simulink library "takeoffToLanding_cl"  (R2018b)
settings: Solver=VariableStepAuto  StartTime=0.0  StopTime=10.0  RelTol=1e-3
undefined symbols (not defined in the file or in its folder): env, FLIGHTCONTROLLER, fltCtrl, initializeBussesFromBlock, maxDeflDns, maxDeflUps, TLSP, vhcl
libraries: filteredPIDController_ul x3, simulink x2, ctrlAllocMatrix_cl x2, dspsigops x1, eulAng2RotMat_ul x1, alphaBeta_ul x1, localApparentWind_ul x1, pathFollowingController_cl x1
settings Model: Creator=jldanie5  LastModifiedBy=jldanie5

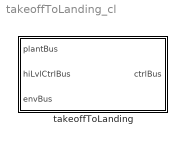
== system takeoffToLanding_cl ==
  takeoffToLanding : Subsystem  LoadFcn=initializeBussesFromBlock(gcb)  InitFcn=initializeBussesFromBlock(gcb)  StartFcn=initializeBussesFromBlock(gcb)  VariantControl=strcmpi(FLIGHTCONTROLLER,'takeoffToLanding')  mask{initPosForInitSStar=vhcl.initPosVecGnd.Value, fluidDensity=env.water.density.Value, pathCtrl=fltCtrl, aeroStruct=vhcl.struct('OCT.aeroSurf')}
      mask prompts: initPosForInitSStar "Initial Position"; fluidDensity "Fluid Density"; pathCtrl "Controller"; aeroStruct "Aerodynamic Structure"
      settings: MinAlgLoopOccurrences=on
      mask DialogControl Container3 Prompt: courseFollow Params
      mask DialogControl Container4 Prompt: setpointToOutput Params

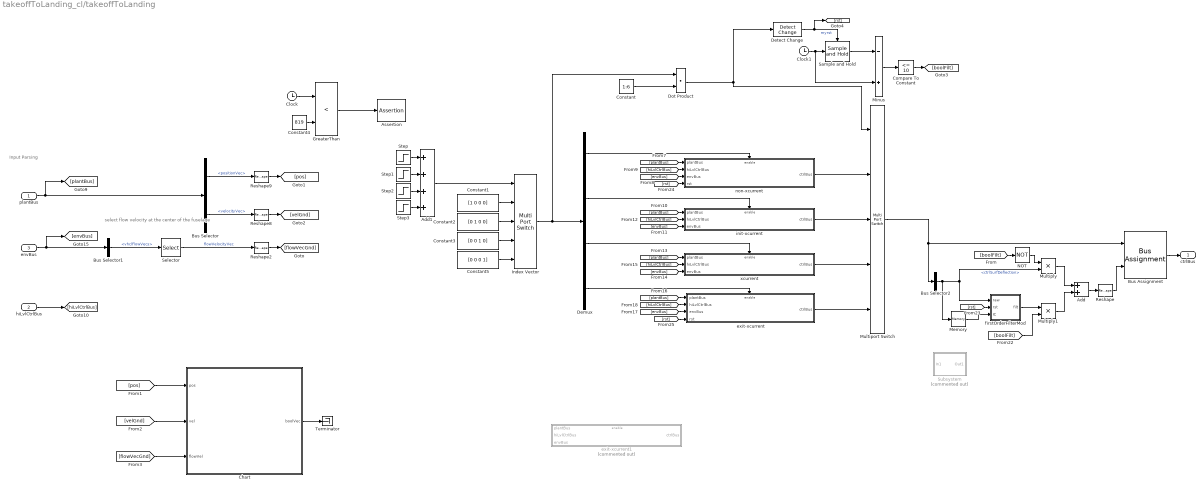
== system takeoffToLanding_cl/takeoffToLanding ==
  note: select flow velocity at the center of the fuselage
  note: Input Parsing
  plantBus : Inport  OutDataTypeStr=Bus: plantBus
  hiLvlCtrlBus : Inport  Port=2  OutDataTypeStr=Bus: hiLvlCtrlBus
  envBus : Inport  Port=3  OutDataTypeStr=Bus: envBus
  Add : Sum
  Add1 : Sum  Inputs=++++
  Assertion : Assertion  Enabled=off  AssertionFailFcn=set_param('OCTModel','SimulationCommand','pause')  StopWhenAssertionFail=off
  Bus Assignment : BusAssignment  AssignedSignals=ctrlSurfDeflection
  Bus Selector : BusSelector  OutputSignals=positionVec,velocityVec
  Bus Selector1 : BusSelector  OutputSignals=vhclFlowVecs
  Bus Selector2 : BusSelector  OutputSignals=ctrlSurfDeflection
  Chart : Stateflow chart  TreatAsAtomicUnit=on
  Clock : Clock
  Clock1 : Clock
  Compare To Constant : simulink/Logic and Bit Operations/Compare To Constant  relop=<=  const=10  OutDataTypeStr=boolean
  Constant : Constant  Value=1:6
  Constant1 : Constant  Value=[1 0 0 0]
  Constant2 : Constant  Value=[0 1 0 0]
  Constant3 : Constant  Value=[0 0 1 0]
  Constant4 : Constant  Value=819
  Constant5 : Constant  Value=[0 0 0 1]
  Demux : Demux
  Detect Change : simulink/Logic and Bit Operations/Detect Change  vinit=0  OutDataTypeStr=boolean
  Dot Product : DotProduct  InputSameDT=on  OutDataTypeStr=Inherit: Inherit via internal rule
  GreaterThan : RelationalOperator  Operator=<  OutDataTypeStr=boolean  RndMeth=Simplest
  Index Vector : MultiPortSwitch  DataPortOrder=Zero-based contiguous  Inputs=4  zeroidx=on
  Memory : Memory  InitialCondition=[0;0;0;0]
  Minus : Sum  Inputs=-+
  Multiply : Product
  Multiply1 : Product
  Multiport Switch : MultiPortSwitch  Inputs=4  DataPortIndices={1,2,3,4,5,6}  DiagnosticForDefault=Warning
  NOT : Logic  Operator=NOT  IconShape=distinctive  AllPortsSameDT=off  OutDataTypeStr=boolean
  Reshape : Reshape
  Reshape2 : Reshape  OutputDimensionality=Column vector (2-D)
  Reshape8 : Reshape  OutputDimensionality=Column vector (2-D)
  Reshape9 : Reshape  OutputDimensionality=Column vector (2-D)
  Sample and Hold : dspsigops/Sample and Hold  trig=Rising edge  initCond=0  latchinput=off
  Selector : Selector  NumberOfDimensions=2  InputPortWidth=3  IndexOptions=Select all,Index vector (dialog)  Indices=[1 3],5  OutputSizes=1,1
  Step : Step  Time=500  SampleTime=0
  Step1 : Step  Time=510  SampleTime=0
  Step2 : Step  Time=800  SampleTime=0
  Step3 : Step  Time=820  After=-3  SampleTime=0
  Subsystem : Subsystem  Commented=on
  Terminator : Terminator
  exit-xcurrent : Subsystem  TreatAsAtomicUnit=on
  exit-xcurrent1 : Subsystem  Commented=on  TreatAsAtomicUnit=on
  "firstOrderFilterMod " : Subsystem  TreatAsAtomicUnit=on  mask{tau=1, ic=0}
      mask prompts: tau "Time Const [s]"; ic "Initial Condition"
      settings: MinAlgLoopOccurrences=on
  init-xcurrent : Subsystem  TreatAsAtomicUnit=on
  non-xcurrent : Subsystem  TreatAsAtomicUnit=on
  xcurrent : Subsystem  TreatAsAtomicUnit=on
  ctrlBus : Outport  OutDataTypeStr=Bus: fltCtrlBus
  wires:
  Constant5/1 -> Index Vector/5
  plantBus/1 -> [plantBus], Bus Selector/1
  Bus Selector/2 -> Reshape8/1  "<velocityVec>"
  Bus Selector/1 -> Reshape9/1  "<positionVec>"
  Reshape2/1 -> [flowVecGnd]
  Reshape8/1 -> [velGnd]
  Reshape9/1 -> [pos]
  Selector/1 -> Reshape2/1  "flowVelocityVec"
  envBus/1 -> [envBus], Bus Selector1/1
  Bus Selector1/1 -> Selector/1  "<vhclFlowVecs>"
  [pos] -> Chart/1(pos)
  [velGnd] -> Chart/2(vel)
  [flowVecGnd] -> Chart/3(flowVel)
  [envBus] -> non-xcurrent/3(envBus)
  [plantBus] -> non-xcurrent/1(plantBus)
  [hiLvlCtrlBus] -> non-xcurrent/2(hiLvlCtrlBus)
  [hiLvlCtrlBus] -> xcurrent/2(hiLvlCtrlBus)
  [plantBus] -> xcurrent/1(plantBus)
  [envBus] -> xcurrent/3(envBus)
  [hiLvlCtrlBus] -> init-xcurrent/2(hiLvlCtrlBus)
  [envBus] -> init-xcurrent/3(envBus)
  [plantBus] -> init-xcurrent/1(plantBus)
  [plantBus] -> exit-xcurrent/1(plantBus)
  [envBus] -> exit-xcurrent/3(envBus)
  [hiLvlCtrlBus] -> exit-xcurrent/2(hiLvlCtrlBus)
  Constant/1 -> Dot Product/2
  Dot Product/1 -> Multiport Switch/1, Detect Change/1
  Chart/1(boolVec) -> Terminator/1
  hiLvlCtrlBus/1 -> [hiLvlCtrlBus]
  Constant1/1 -> Index Vector/2
  Constant2/1 -> Index Vector/3
  Constant3/1 -> Index Vector/4
  Clock/1 -> GreaterThan/1
  Constant4/1 -> GreaterThan/2
  GreaterThan/1 -> Assertion/1
  Add1/1 -> Index Vector/1
  Index Vector/1 -> Dot Product/1, Demux/1
  Clock1/1 -> Minus/2, Sample and Hold/1
  Detect Change/1 -> [rst], Sample and Hold/Trigger  "myrst"
  Sample and Hold/1 -> Minus/1
  Minus/1 -> Compare To Constant/1
  Compare To Constant/1 -> [boolFilt]
  Bus Assignment/1 -> ctrlBus/1
  Multiport Switch/1 -> Bus Selector2/1, Bus Assignment/1
  Bus Selector2/1 -> Multiply/2, "firstOrderFilterMod "/1(raw), Memory/1  "<ctrlSurfDeflection>"
  [boolFilt] -> NOT/1
  NOT/1 -> Multiply/1
  "firstOrderFilterMod "/1(filt) -> Multiply1/1
  [boolFilt] -> Multiply1/2
  [rst] -> "firstOrderFilterMod "/2(rst)
  Multiply/1 -> Add/1
  Multiply1/1 -> Add/2
  Add/1 -> Reshape/1
  Reshape/1 -> Bus Assignment/2
  Memory/1 -> "firstOrderFilterMod "/3(IC)
  Step/1 -> Add1/1
  Step1/1 -> Add1/2
  Step2/1 -> Add1/3
  Step3/1 -> Add1/4
  [rst] -> non-xcurrent/4("rst ")
  [rst] -> exit-xcurrent/4(rst)
  exit-xcurrent/1(ctrlBus) -> Multiport Switch/5
  xcurrent/1(ctrlBus) -> Multiport Switch/4
  init-xcurrent/1(ctrlBus) -> Multiport Switch/3
  non-xcurrent/1(ctrlBus) -> Multiport Switch/2
  Demux/1 -> non-xcurrent/Enable
  Demux/2 -> init-xcurrent/Enable
  Demux/3 -> xcurrent/Enable
  Demux/4 -> exit-xcurrent/Enable

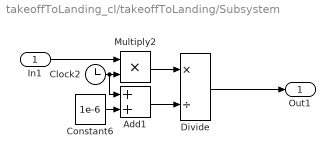
== system takeoffToLanding_cl/takeoffToLanding/Subsystem ==
  In1 : Inport
  Add1 : Sum
  Clock2 : Clock
  Constant6 : Constant  Value=1e-6
  Divide : Product  Inputs=*/
  Multiply2 : Product
  Out1 : Outport
  wires:
  In1/1 -> Multiply2/1
  Constant6/1 -> Add1/2
  Clock2/1 -> Add1/1, Multiply2/2
  Divide/1 -> Out1/1
  Multiply2/1 -> Divide/1
  Add1/1 -> Divide/2

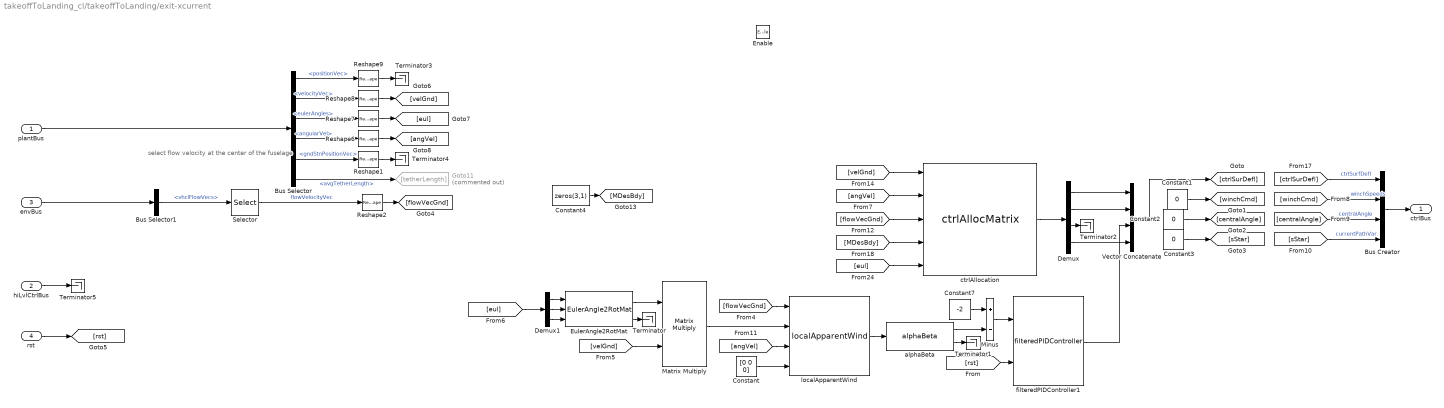
== system takeoffToLanding_cl/takeoffToLanding/exit-xcurrent ==
  note: select flow velocity at the center of the fuselage
  plantBus : Inport  OutDataTypeStr=Bus: plantBus
  hiLvlCtrlBus : Inport  Port=2  OutDataTypeStr=Bus: hiLvlCtrlBus
  envBus : Inport  Port=3  OutDataTypeStr=Bus: envBus
  rst : Inport  Port=4
  Enable : EnablePort
  Bus Creator : BusCreator  Inputs=4  OutDataTypeStr=Bus: fltCtrlBus
      settings: InheritFromInputs=off
  Bus Selector : BusSelector  OutputSignals=positionVec,velocityVec,eulerAngles,angularVel,gndStnPositionVec,avgTetherLength
  Bus Selector1 : BusSelector  OutputSignals=vhclFlowVecs
  Constant : Constant  Value=[0 0 0]
  Constant1 : Constant  Value=0
  Constant2 : Constant  Value=0
  Constant3 : Constant  Value=0
  Constant4 : Constant  Value=zeros(3,1)
  Constant7 : Constant  Value=-2
  Demux : Demux
  Demux1 : Demux  Outputs=3
  EulerAngle2RotMat : eulAng2RotMat_ul/EulerAngle2RotMat  SystemSampleTime=-1
  Goto11 : Goto  Commented=on  GotoTag=tetherLength
  Matrix Multiply : Product  Multiplication=Matrix(*)
  Minus : Sum  Inputs=+-
  Reshape{1..2,6..9} (6 alike) : Reshape  OutputDimensionality=Column vector (2-D)
  Selector : Selector  NumberOfDimensions=2  InputPortWidth=3  IndexOptions=Select all,Index vector (dialog)  Indices=[1 3],5  OutputSizes=1,1
  Terminator{,1..5} (6 alike) : Terminator
  Vector Concatenate : Concatenate  NumInputs=4
  alphaBeta : alphaBeta_ul/alphaBeta  SystemSampleTime=-1
  ctrlAllocation : ctrlAllocMatrix_cl/ctrlAllocMatrix  aeroStruct=aeroStruct  fluidDensity=fluidDensity  ctrlUpMax=pathCtrl.controlSigMax.upperLimit.Value  ctrlDnMax=pathCtrl.controlSigMax.lowerLimit.Value
  filteredPIDController1 : filteredPIDController_ul/filteredPIDController  kp=kpElev  ki=kiElev  kd=kdElev  Value=.01  externalReset=rising
  localApparentWind : localApparentWind_ul/localApparentWind  SystemSampleTime=-1
  ctrlBus : Outport  OutDataTypeStr=Bus: fltCtrlBus
  wires:
  [sStar] -> Bus Creator/4  "currentPathVar"
  [ctrlSurDefl] -> Bus Creator/1  "ctrlSurfDefl"
  [winchCmd] -> Bus Creator/2  "winchSpeeds"
  Bus Creator/1 -> ctrlBus/1
  [centralAngle] -> Bus Creator/3  "centralAngle"
  Constant1/1 -> [winchCmd]
  Constant2/1 -> [centralAngle]
  Constant3/1 -> [sStar]
  Bus Selector/1 -> Reshape9/1  "<positionVec>"
  Bus Selector/3 -> Reshape7/1  "<eulerAngles>"
  Bus Selector/2 -> Reshape8/1  "<velocityVec>"
  Reshape7/1 -> [eul]
  Bus Selector/4 -> Reshape6/1  "<angularVel>"
  Reshape8/1 -> [velGnd]
  Selector/1 -> Reshape2/1  "flowVelocityVec"
  Reshape9/1 -> Terminator3/1
  Bus Selector/5 -> Reshape1/1  "<gndStnPositionVec>"
  Reshape2/1 -> [flowVecGnd]
  Bus Selector1/1 -> Selector/1  "<vhclFlowVecs>"
  envBus/1 -> Bus Selector1/1
  Reshape1/1 -> Terminator4/1
  plantBus/1 -> Bus Selector/1
  Reshape6/1 -> [angVel]
  [flowVecGnd] -> ctrlAllocation/3
  [angVel] -> ctrlAllocation/2
  [eul] -> ctrlAllocation/5
  [MDesBdy] -> ctrlAllocation/4
  [velGnd] -> ctrlAllocation/1
  Bus Selector/6 -> Goto11/1  "<avgTetherLength>"
  ctrlAllocation/1 -> Demux/1
  Vector Concatenate/1 -> [ctrlSurDefl]
  Minus/1 -> filteredPIDController1/1
  Demux/1 -> Vector Concatenate/1
  Demux/2 -> Vector Concatenate/2
  Demux/4 -> Vector Concatenate/4
  localApparentWind/1 -> alphaBeta/1
  [flowVecGnd] -> localApparentWind/1
  Demux1/1 -> EulerAngle2RotMat/1
  Demux1/2 -> EulerAngle2RotMat/2
  Demux1/3 -> EulerAngle2RotMat/3
  [eul] -> Demux1/1
  EulerAngle2RotMat/1 -> Matrix Multiply/1
  [velGnd] -> Matrix Multiply/2
  EulerAngle2RotMat/2 -> Terminator/1
  Matrix Multiply/1 -> localApparentWind/2
  [angVel] -> localApparentWind/3
  Constant/1 -> localApparentWind/4
  Constant7/1 -> Minus/1
  alphaBeta/1 -> Minus/2
  filteredPIDController1/1 -> Vector Concatenate/3
  Demux/3 -> Terminator2/1
  alphaBeta/2 -> Terminator1/1
  Constant4/1 -> [MDesBdy]
  hiLvlCtrlBus/1 -> Terminator5/1
  rst/1 -> [rst]
  [rst] -> filteredPIDController1/2

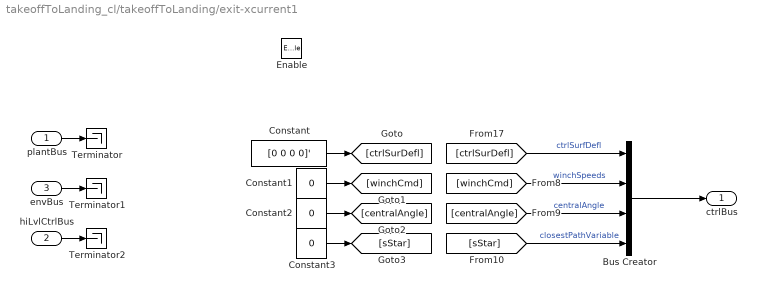
== system takeoffToLanding_cl/takeoffToLanding/exit-xcurrent1 ==
  plantBus : Inport  OutDataTypeStr=Bus: plantBus
  hiLvlCtrlBus : Inport  Port=2  OutDataTypeStr=Bus: hiLvlCtrlBus
  envBus : Inport  Port=3  OutDataTypeStr=Bus: envBus
  Enable : EnablePort
  Bus Creator : BusCreator  Inputs=4  OutDataTypeStr=Bus: fltCtrlBus
      settings: InheritFromInputs=off
  Constant : Constant  Value=[0 0 0 0]'
  Constant1 : Constant  Value=0
  Constant2 : Constant  Value=0
  Constant3 : Constant  Value=0
  Terminator : Terminator
  Terminator1 : Terminator
  Terminator2 : Terminator
  ctrlBus : Outport  OutDataTypeStr=Bus: fltCtrlBus
  wires:
  [ctrlSurDefl] -> Bus Creator/1  "ctrlSurfDefl"
  [centralAngle] -> Bus Creator/3  "centralAngle"
  [winchCmd] -> Bus Creator/2  "winchSpeeds"
  envBus/1 -> Terminator1/1
  hiLvlCtrlBus/1 -> Terminator2/1
  Constant2/1 -> [centralAngle]
  plantBus/1 -> Terminator/1
  [sStar] -> Bus Creator/4  "closestPathVariable"
  Constant1/1 -> [winchCmd]
  Bus Creator/1 -> ctrlBus/1
  Constant3/1 -> [sStar]
  Constant/1 -> [ctrlSurDefl]

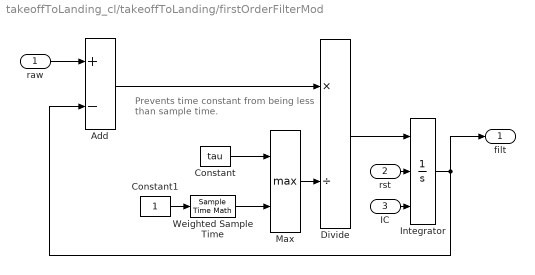
== system takeoffToLanding_cl/takeoffToLanding/firstOrderFilterMod  ==
  note: Prevents time constant from
      | being less than sample time.
  raw : Inport
  rst : Inport  Port=2
  IC : Inport  Port=3
  Add : Sum  Inputs=+-
  Constant : Constant  Value=tau
  Constant1 : Constant
  Divide : Product  Inputs=*/
  Integrator : Integrator  ExternalReset=rising  InitialConditionSource=external  InitialCondition=ic
  Max : MinMax  Function=max  Inputs=2
  Weighted Sample Time : SampleTimeMath  TsampMathOp=Ts Only
  filt : Outport
  wires:
  raw/1 -> Add/1
  Add/1 -> Divide/1
  Max/1 -> Divide/2
  Constant/1 -> Max/1
  Constant1/1 -> Weighted Sample Time/1
  Weighted Sample Time/1 -> Max/2
  Divide/1 -> Integrator/1
  Integrator/1 -> Add/2, filt/1
  IC/1 -> Integrator/3
  rst/1 -> Integrator/2

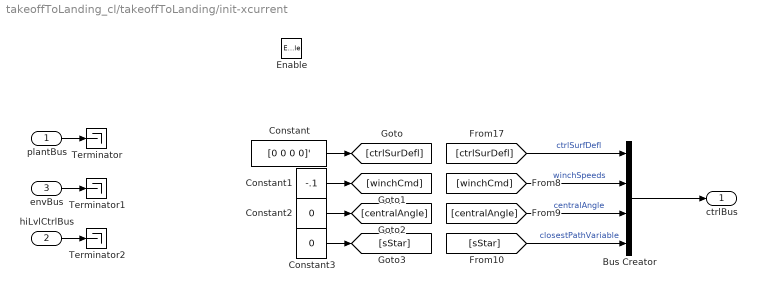
== system takeoffToLanding_cl/takeoffToLanding/init-xcurrent ==
  plantBus : Inport  OutDataTypeStr=Bus: plantBus
  hiLvlCtrlBus : Inport  Port=2  OutDataTypeStr=Bus: hiLvlCtrlBus
  envBus : Inport  Port=3  OutDataTypeStr=Bus: envBus
  Enable : EnablePort
  Bus Creator : BusCreator  Inputs=4  OutDataTypeStr=Bus: fltCtrlBus
      settings: InheritFromInputs=off
  Constant : Constant  Value=[0 0 0 0]'
  Constant1 : Constant  Value=-.1
  Constant2 : Constant  Value=0
  Constant3 : Constant  Value=0
  Terminator : Terminator
  Terminator1 : Terminator
  Terminator2 : Terminator
  ctrlBus : Outport  OutDataTypeStr=Bus: fltCtrlBus
  wires:
  [ctrlSurDefl] -> Bus Creator/1  "ctrlSurfDefl"
  [centralAngle] -> Bus Creator/3  "centralAngle"
  [winchCmd] -> Bus Creator/2  "winchSpeeds"
  envBus/1 -> Terminator1/1
  hiLvlCtrlBus/1 -> Terminator2/1
  Constant2/1 -> [centralAngle]
  plantBus/1 -> Terminator/1
  [sStar] -> Bus Creator/4  "closestPathVariable"
  Constant1/1 -> [winchCmd]
  Bus Creator/1 -> ctrlBus/1
  Constant3/1 -> [sStar]
  Constant/1 -> [ctrlSurDefl]

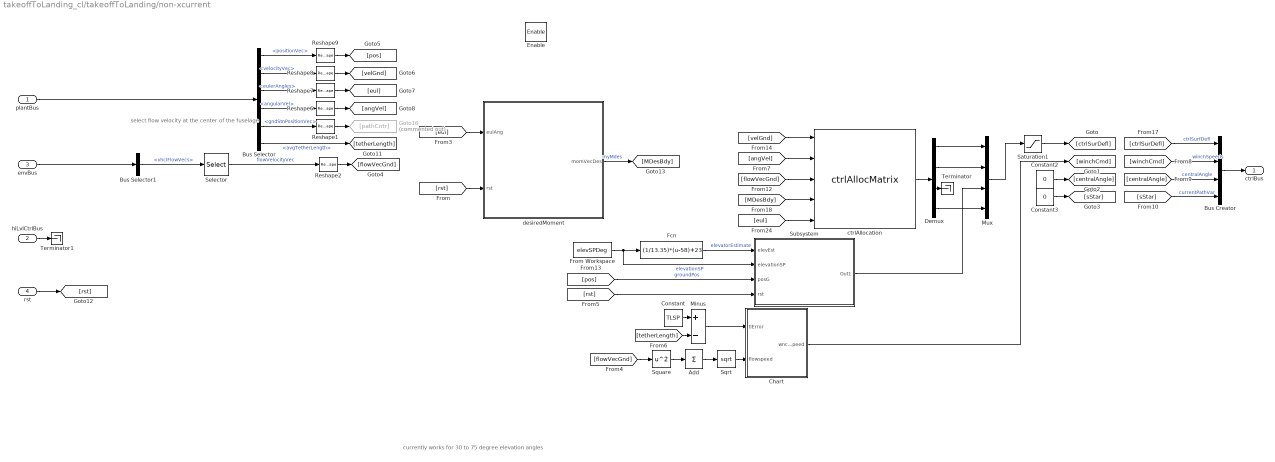
== system takeoffToLanding_cl/takeoffToLanding/non-xcurrent ==
  note: select flow velocity at the center of the fuselage
  note: currently works for 30 to 75 degree elevation angles
  plantBus : Inport  OutDataTypeStr=Bus: plantBus
  hiLvlCtrlBus : Inport  Port=2  OutDataTypeStr=Bus: hiLvlCtrlBus
  envBus : Inport  Port=3  OutDataTypeStr=Bus: envBus
  "rst " : Inport  Port=4
  Enable : EnablePort
  Add : Sum  Inputs=+
  Bus Creator : BusCreator  Inputs=4  OutDataTypeStr=Bus: fltCtrlBus
      settings: InheritFromInputs=off
  Bus Selector : BusSelector  OutputSignals=positionVec,velocityVec,eulerAngles,angularVel,gndStnPositionVec,avgTetherLength
  Bus Selector1 : BusSelector  OutputSignals=vhclFlowVecs
  Chart : Stateflow chart  TreatAsAtomicUnit=on
  Constant : Constant  Value=TLSP
  Constant2 : Constant  Value=0
  Constant3 : Constant  Value=0
  Demux : Demux
  Fcn : Fcn  Expr=(1/13.35)*(u-58)+23
  From Workspace : FromWorkspace  VariableName=elevSPDeg  SampleTime=0
  Goto16 : Goto  Commented=on  GotoTag=pathCntr
  Minus : Sum  Inputs=+-
  Mux : Mux
  Reshape{1..2,6..9} (6 alike) : Reshape  OutputDimensionality=Column vector (2-D)
  Saturation1 : Saturate  UpperLimit=maxDeflUps  LowerLimit=maxDeflDns
  Selector : Selector  NumberOfDimensions=2  InputPortWidth=3  IndexOptions=Select all,Index vector (dialog)  Indices=[1 3],5  OutputSizes=1,1
  Sqrt : Sqrt  SaturateOnIntegerOverflow=on
  Square : Math  Operator=square  SaturateOnIntegerOverflow=on
  Subsystem : Subsystem
  Terminator : Terminator
  Terminator1 : Terminator
  ctrlAllocation : ctrlAllocMatrix_cl/ctrlAllocMatrix  aeroStruct=aeroStruct  fluidDensity=fluidDensity  ctrlUpMax=pathCtrl.controlSigMax.upperLimit.Value  ctrlDnMax=pathCtrl.controlSigMax.lowerLimit.Value
  desiredMoment : Subsystem
  ctrlBus : Outport  OutDataTypeStr=Bus: fltCtrlBus
  wires:
  [sStar] -> Bus Creator/4  "currentPathVar"
  [ctrlSurDefl] -> Bus Creator/1  "ctrlSurfDefl"
  [winchCmd] -> Bus Creator/2  "winchSpeeds"
  Bus Creator/1 -> ctrlBus/1
  [centralAngle] -> Bus Creator/3  "centralAngle"
  Chart/1(wnchspeed) -> [winchCmd]
  Constant2/1 -> [centralAngle]
  Constant3/1 -> [sStar]
  desiredMoment/1(momVecDes) -> [MDesBdy]  "myMdes"
  Bus Selector/1 -> Reshape9/1  "<positionVec>"
  Bus Selector/3 -> Reshape7/1  "<eulerAngles>"
  Bus Selector/2 -> Reshape8/1  "<velocityVec>"
  Reshape7/1 -> [eul]
  Bus Selector/4 -> Reshape6/1  "<angularVel>"
  Reshape8/1 -> [velGnd]
  Selector/1 -> Reshape2/1  "flowVelocityVec"
  Reshape9/1 -> [pos]
  Bus Selector/5 -> Reshape1/1  "<gndStnPositionVec>"
  Reshape2/1 -> [flowVecGnd]
  Bus Selector1/1 -> Selector/1  "<vhclFlowVecs>"
  envBus/1 -> Bus Selector1/1
  Reshape1/1 -> Goto16/1
  plantBus/1 -> Bus Selector/1
  Reshape6/1 -> [angVel]
  [eul] -> desiredMoment/1(eulAng)
  [flowVecGnd] -> ctrlAllocation/3
  [angVel] -> ctrlAllocation/2
  [eul] -> ctrlAllocation/5
  [MDesBdy] -> ctrlAllocation/4
  [velGnd] -> ctrlAllocation/1
  [flowVecGnd] -> Square/1
  Add/1 -> Sqrt/1
  Bus Selector/6 -> [tetherLength]  "<avgTetherLength>"
  Constant/1 -> Minus/1
  Minus/1 -> Chart/1(tlError)
  [tetherLength] -> Minus/2
  Sqrt/1 -> Chart/2(flowspeed)
  Square/1 -> Add/1
  ctrlAllocation/1 -> Demux/1
  Demux/1 -> Mux/1
  Demux/2 -> Mux/2
  Demux/4 -> Mux/4
  Demux/3 -> Terminator/1
  Mux/1 -> Saturation1/1
  From Workspace/1 -> Fcn/1, Subsystem/2(elevationSP)  "elevationSP"
  Fcn/1 -> Subsystem/1(elevEst)  "elevatorEstimate"
  [pos] -> Subsystem/3(posG)  "groundPos"
  Subsystem/1(Out1) -> Mux/3
  "rst "/1 -> [rst]
  [rst] -> Subsystem/4("rst ")
  hiLvlCtrlBus/1 -> Terminator1/1
  [rst] -> desiredMoment/2(rst)
  Saturation1/1 -> [ctrlSurDefl]

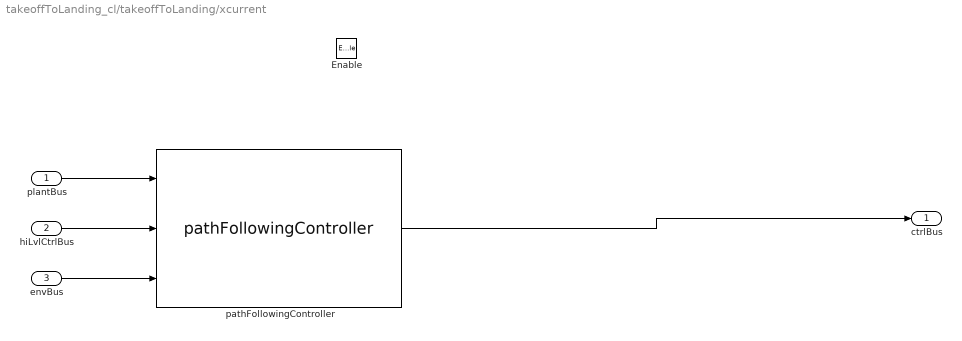
== system takeoffToLanding_cl/takeoffToLanding/xcurrent ==
  plantBus : Inport  OutDataTypeStr=Bus: plantBus
  hiLvlCtrlBus : Inport  Port=2  OutDataTypeStr=Bus: hiLvlCtrlBus
  envBus : Inport  Port=3  OutDataTypeStr=Bus: envBus
  Enable : EnablePort
  pathFollowingController : pathFollowingController_cl/pathFollowingController  VariantControl=strcmpi(FLIGHTCONTROLLER,'pathFollowingController')  initPosForInitSStar=vhcl.initPosVecGnd.Value  fluidDensity=env.water.density.Value  pathCtrl=fltCtrl  aeroStruct=vhcl.struct('OCT.aeroSurf')
  ctrlBus : Outport  OutDataTypeStr=Bus: fltCtrlBus
  wires:
  plantBus/1 -> pathFollowingController/1
  hiLvlCtrlBus/1 -> pathFollowingController/2
  envBus/1 -> pathFollowingController/3
  pathFollowingController/1 -> ctrlBus/1

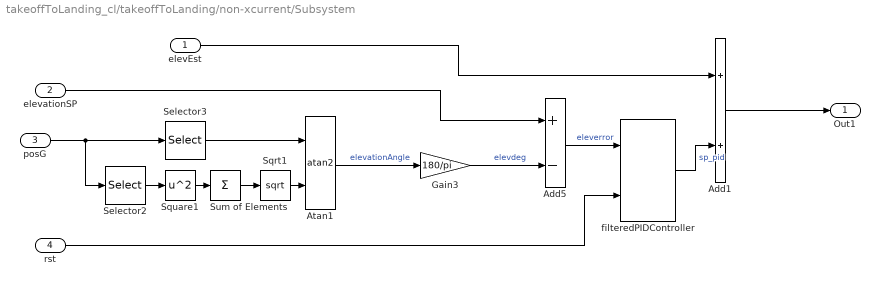
== system takeoffToLanding_cl/takeoffToLanding/non-xcurrent/Subsystem ==
  elevEst : Inport
  elevationSP : Inport  Port=2
  posG : Inport  Port=3
  "rst " : Inport  Port=4
  Add1 : Sum
  Add5 : Sum  Inputs=+-
  Atan1 : Trigonometry  Operator=atan2
  Gain3 : Gain  Gain=180/pi
  Selector2 : Selector  InputPortWidth=3  IndexOptions=Index vector (dialog)  Indices=[1 2]  OutputSizes=1
  Selector3 : Selector  InputPortWidth=3  IndexOptions=Index vector (dialog)  Indices=3  OutputSizes=1
  Sqrt1 : Sqrt  SaturateOnIntegerOverflow=on
  Square1 : Math  Operator=square  SaturateOnIntegerOverflow=on
  Sum of Elements : Sum  Inputs=+
  filteredPIDController : filteredPIDController_ul/filteredPIDController  kp=kpElev  ki=kiElev  kd=kdElev  Value=.01  externalReset=rising
  Out1 : Outport
  wires:
  posG/1 -> Selector2/1, Selector3/1
  Square1/1 -> Sum of Elements/1
  Selector2/1 -> Square1/1
  Gain3/1 -> Add5/2  "elevdeg"
  filteredPIDController/1 -> Add1/2  "sp_pid"
  Sqrt1/1 -> Atan1/2
  Selector3/1 -> Atan1/1
  Atan1/1 -> Gain3/1  "elevationAngle"
  Sum of Elements/1 -> Sqrt1/1
  Add5/1 -> filteredPIDController/1  "eleverror"
  Add1/1 -> Out1/1
  elevEst/1 -> Add1/1
  elevationSP/1 -> Add5/1
  "rst "/1 -> filteredPIDController/2

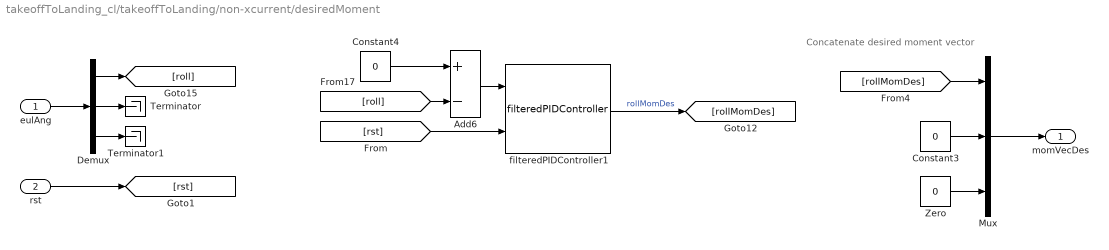
== system takeoffToLanding_cl/takeoffToLanding/non-xcurrent/desiredMoment ==
  note: Concatenate desired moment vector
  eulAng : Inport
  rst : Inport  Port=2
  Add6 : Sum  Inputs=+-
  Constant3 : Constant  Value=0
  Constant4 : Constant  Value=0
  Demux : Demux  Outputs=3
  Mux : Mux  Inputs=3
  Terminator : Terminator
  Terminator1 : Terminator
  Zero : Constant  Value=0  OutDataTypeStr=Inherit: Inherit via back propagation
  filteredPIDController1 : filteredPIDController_ul/filteredPIDController  kp=pathCtrl.rollMoment.kp.Value  ki=0  kd=pathCtrl.rollMoment.kd.Value  Value=pathCtrl.rollMoment.tau.Value  externalReset=rising
  momVecDes : Outport
  wires:
  Zero/1 -> Mux/3
  [rollMomDes] -> Mux/1
  Constant3/1 -> Mux/2
  Mux/1 -> momVecDes/1
  Demux/1 -> [roll]
  eulAng/1 -> Demux/1
  filteredPIDController1/1 -> [rollMomDes]  "rollMomDes"
  Add6/1 -> filteredPIDController1/1
  [roll] -> Add6/2
  Constant4/1 -> Add6/1
  Demux/2 -> Terminator/1
  Demux/3 -> Terminator1/1
  rst/1 -> [rst]
  [rst] -> filteredPIDController1/2

== stateflow chart takeoffToLanding_cl/takeoffToLanding/Chart ==
  state Default
    boolVec=[0 1 0 0 0 0];
  (default) -> Default
  data: boolVec output; pos input; vel input; flowVel input

== stateflow chart takeoffToLanding_cl/takeoffToLanding/non-xcurrent/Chart ==
  state %Spool In
    wnchspeed=-flowspeed*.2;
  state %Spool out
    wnchspeed=flowspeed*.2;
  state %Correct
    wnchspeed=0;
  (default) -> %Spool out
  %Correct -> %Spool In [order 1] : [tlError<-1]
  %Spool out -> %Correct : [abs(tlError)<.5]
  %Spool In -> %Correct : [abs(tlError)<.5]
  %Correct -> %Spool out [order 2] : [tlError>1]
  data: tlError input; wnchspeed output; flowspeed input
